simulink library "Enx_PWMx_to_TxHL"  (R2014b)
settings: Solver=ode45  StartTime=0.0  StopTime=10.0  RelTol=1e-3
settings Model: Creator=vda2sh  LastModifiedBy=vda2sh

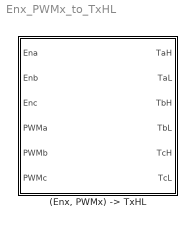
== system Enx_PWMx_to_TxHL ==
  "(Enx, PWMx) -> TxHL" : Subsystem
      mask help: This block computes the single transistor control signals `TxH` respectively `TxL` from the `Enx` and `PWMx` signals, with x in {a, b, c}.
      mask Help: Block with beta-status, actual no documentation.
      mask Display:
      | text(0.6, 0.15, 'beta')
      | port_label('input',1,'Ena [-]')
      | port_label('input',2,'Enb [-]')
      | port_label('input',3,'Enc [-]')
      | port_label('input',4,'PWMa [-]')
      | port_label('input',5,'PWMb [-]')
      | port_label('input',6,'PWMc [-]')
      | port_label('output',1,'TaH [-]')
      | port_label('output',2,'TaL [-]')
      | port_label('output',3,'TbH [-]')
      | port_label('output',4,'TbL [-]')
      | port_label('output',5,'TcH [-]')
      | port_label('output',6,'TcL [-]')

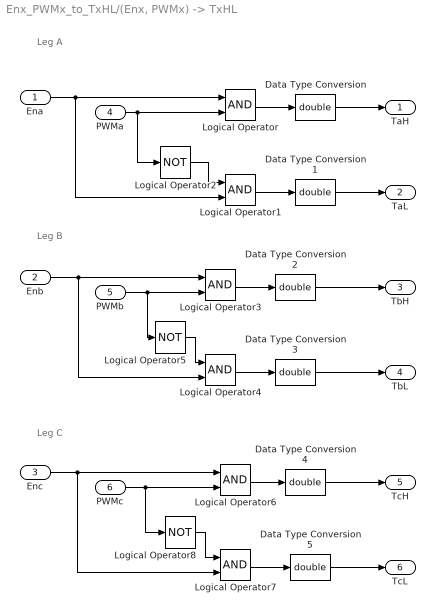
== system Enx_PWMx_to_TxHL/(Enx, PWMx) -> TxHL ==
  note: Leg B
  note: Leg A
  note: Leg C
  Ena : Inport
  Enb : Inport  Port=2
  Enc : Inport  Port=3
  PWMa : Inport  Port=4
  PWMb : Inport  Port=5
  PWMc : Inport  Port=6
  Data Type Conversion{,1..5} (6 alike) : DataTypeConversion  OutDataTypeStr=double
  Logical Operator{,1,3..4,6..7} (6 alike) : Logic  AllPortsSameDT=off  OutDataTypeStr=boolean
  Logical Operator2 : Logic  Operator=NOT  AllPortsSameDT=off  OutDataTypeStr=boolean
  Logical Operator5 : Logic  Operator=NOT  AllPortsSameDT=off  OutDataTypeStr=boolean
  Logical Operator8 : Logic  Operator=NOT  AllPortsSameDT=off  OutDataTypeStr=boolean
  TaH : Outport
  TaL : Outport  Port=2
  TbH : Outport  Port=3
  TbL : Outport  Port=4
  TcH : Outport  Port=5
  TcL : Outport  Port=6
  wires:
  PWMa/1 -> Logical Operator2/1, Logical Operator/2
  Logical Operator/1 -> Data Type Conversion/1
  Logical Operator1/1 -> Data Type Conversion1/1
  Ena/1 -> Logical Operator/1, Logical Operator1/2
  PWMb/1 -> Logical Operator5/1, Logical Operator3/2
  Enb/1 -> Logical Operator4/2, Logical Operator3/1
  Logical Operator3/1 -> Data Type Conversion2/1
  Logical Operator4/1 -> Data Type Conversion3/1
  PWMc/1 -> Logical Operator8/1, Logical Operator6/2
  Enc/1 -> Logical Operator7/2, Logical Operator6/1
  Logical Operator6/1 -> Data Type Conversion4/1
  Logical Operator7/1 -> Data Type Conversion5/1
  Data Type Conversion/1 -> TaH/1
  Data Type Conversion1/1 -> TaL/1
  Data Type Conversion2/1 -> TbH/1
  Data Type Conversion3/1 -> TbL/1
  Data Type Conversion4/1 -> TcH/1
  Data Type Conversion5/1 -> TcL/1
  Logical Operator2/1 -> Logical Operator1/1
  Logical Operator5/1 -> Logical Operator4/1
  Logical Operator8/1 -> Logical Operator7/1
